simulink model "TaskOverrunTest"  (R2018b)
settings: Solver=FixedStepAuto  StartTime=0.0  StopTime=inf  FixedStep=0.005  RelTol=1e-3
libraries: BrickPi x14
settings Model: SimulationMode=external  Creator=Isshu  LastModifiedBy=Isshu
settings SolverCC: PositivePriorityOrder=on
settings OptimizationCC: EnhancedBackFolding=on  PassReuseOutputArgsAs=Individual arguments  MaxStackSize=64  OptimizeBlockOrder=speed  DifferentSizesBufferReuse=on  OptimizationCustomize=off
settings DebuggingCC: ParameterTunabilityLossMsg=error
settings HardwareCC: ProdBitPerPointer=32  ProdBitPerSizeT=32  ProdBitPerPtrDiffT=32  ProdLargestAtomicInteger=Long  ProdLargestAtomicFloat=Double  ProdWordSize=32  ProdHWDeviceType=ARM Compatible->ARM Cortex  UseEmbeddedCoderFeatures=off  UseSimulinkCoderFeatures=off
settings SFSimCC: MATLABDynamicMemAlloc=off
settings RTWCC: SystemTargetFile=ert.tlc  HardwareBoard=Raspberry Pi  TLCOptions="-aInlineSetEventsForThisBaseRateFcn=TLC_FALSE -aSuppressMultiTaskScheduler=TLC_FALSE  -aRateBasedStepFcn=0"  TemplateMakefile=ert_default_tmf  GenerateReport=on  Toolchain=GNU GCC Raspberry Pi  BuildConfiguration=Faster Runs  IncludeHyperlinkInReport=on  LaunchReport=on  GenerateTraceInfo=on  GenerateTraceReport=on  GenerateTraceReportSl=on  GenerateTraceReportSf=on  GenerateTraceReportEml=on
settings CodeAppCC: ForceParamTrailComments=on  IgnoreCustomStorageClasses=off  OperatorAnnotations=on  SimulinkDataObjDesc=on  SFDataObjDesc=on  MangleLength=10  InsertBlockDesc=on
settings ERTTargetCC: SupportNonInlinedSFcns=on  SupportVariableSizeSignals=on

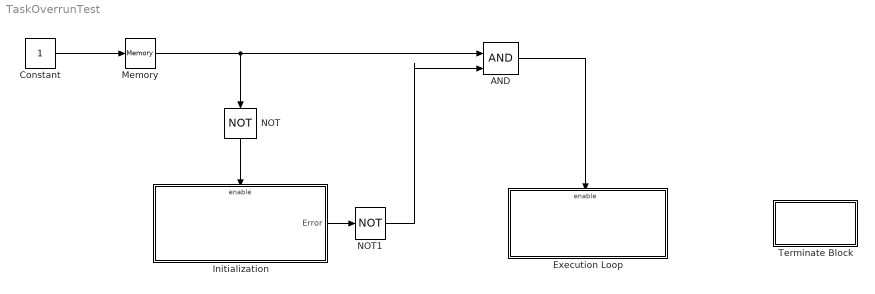
== system TaskOverrunTest ==
  AND : Logic  IconShape=distinctive  AllPortsSameDT=off  OutDataTypeStr=boolean
  Constant : Constant
  Execution Loop : Subsystem
  Initialization : Subsystem  TreatAsAtomicUnit=on
  Memory : Memory
  NOT : Logic  Operator=NOT  IconShape=distinctive  AllPortsSameDT=off  OutDataTypeStr=boolean
  NOT1 : Logic  Operator=NOT  IconShape=distinctive  AllPortsSameDT=off  OutDataTypeStr=boolean
  Terminate Block : Subsystem  TreatAsAtomicUnit=on
  wires:
  Constant/1 -> Memory/1
  NOT/1 -> Initialization/Enable
  Memory/1 -> AND/1, NOT/1
  Initialization/1(Error) -> NOT1/1
  AND/1 -> Execution Loop/Enable
  NOT1/1 -> AND/2

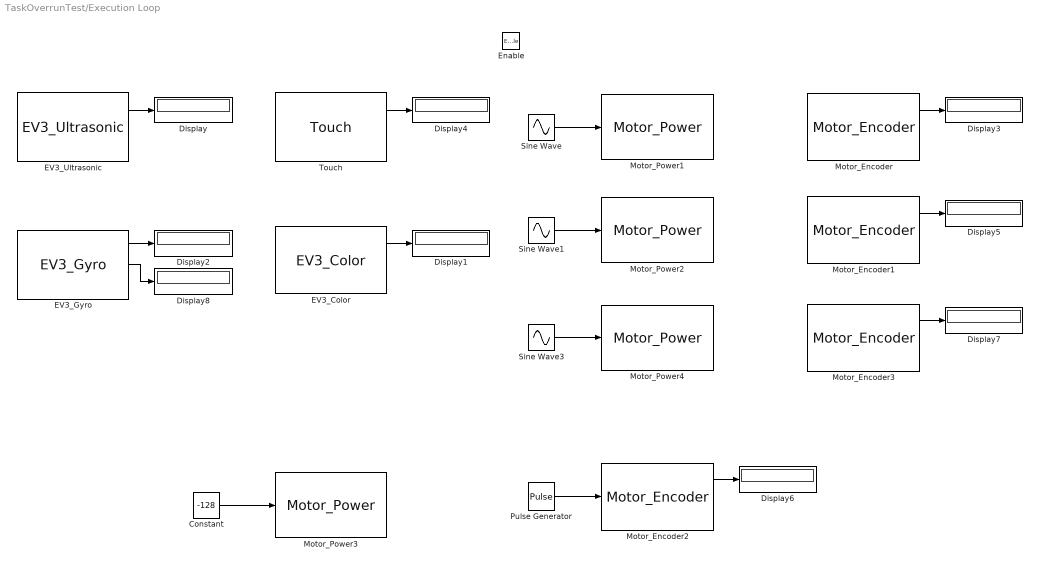
== system TaskOverrunTest/Execution Loop ==
  Enable : EnablePort
  Constant : Constant  Value=-128
  Display{,1..8} (9 alike) : Display
  EV3_Color : BrickPi/EV3_Color  SensorPort=4  SensorType=SENSOR_TYPE_EV3_COLOR_REFLECTED
  EV3_Gyro : BrickPi/EV3_Gyro  SensorPort=3  SensorType=SENSOR_TYPE_EV3_GYRO_ABS_DPS
  EV3_Ultrasonic : BrickPi/EV3_Ultrasonic  SensorPort=1  SensorType=SENSOR_TYPE_EV3_ULTRASONIC_CM
  Motor_Encoder : BrickPi/Motor_Encoder  MotorPort=A  ResetMode=Never reset
  Motor_Encoder1 : BrickPi/Motor_Encoder  MotorPort=B  ResetMode=Never reset
  Motor_Encoder2 : BrickPi/Motor_Encoder  MotorPort=C  ResetMode=Reset on external signal
  Motor_Encoder3 : BrickPi/Motor_Encoder  MotorPort=D  ResetMode=Never reset
  Motor_Power1 : BrickPi/Motor_Power  MotorPort=A  choice=Power  Kp=0  Kd=0
  Motor_Power2 : BrickPi/Motor_Power  MotorPort=B  choice=Power  Kp=0  Kd=0
  Motor_Power3 : BrickPi/Motor_Power  MotorPort=C  choice=Power  Kp=0  Kd=0
  Motor_Power4 : BrickPi/Motor_Power  MotorPort=D  choice=Power  Kp=0  Kd=0
  Pulse Generator : DiscretePulseGenerator  PulseType=Time based  Period=5
  Sine Wave : Sin  Amplitude=10  SampleTime=0
  Sine Wave1 : Sin  Amplitude=10  SampleTime=0
  Sine Wave3 : Sin  Amplitude=10  SampleTime=0
  Touch : BrickPi/Touch  SensorPort=2  SensorType=SENSOR_TYPE_TOUCH_EV3
  wires:
  Sine Wave1/1 -> Motor_Power2/1
  Sine Wave3/1 -> Motor_Power4/1
  EV3_Gyro/1 -> Display2/1
  Constant/1 -> Motor_Power3/1
  Motor_Encoder/1 -> Display3/1
  EV3_Ultrasonic/1 -> Display/1
  Motor_Encoder2/1 -> Display6/1
  Sine Wave/1 -> Motor_Power1/1
  Touch/1 -> Display4/1
  Motor_Encoder1/1 -> Display5/1
  EV3_Color/1 -> Display1/1
  Motor_Encoder3/1 -> Display7/1
  EV3_Gyro/2 -> Display8/1
  Pulse Generator/1 -> Motor_Encoder2/1

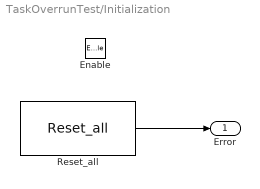
== system TaskOverrunTest/Initialization ==
  Enable : EnablePort
  Reset_all : BrickPi/Reset_all  SystemSampleTime=-1
  Error : Outport
  wires:
  Reset_all/1 -> Error/1

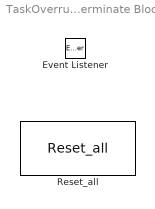
== system TaskOverrunTest/Terminate Block ==
  Event Listener : EventListener  DisableCoverage=on  EventType=Terminate  EventName=reset
  Reset_all : BrickPi/Reset_all  SystemSampleTime=-1
